simulink model "sandip_MIL_SIL"  (R2019b)
settings: Solver=FixedStepDiscrete  StartTime=0.0  StopTime=16  FixedStep=1  RelTol=1e-3
values from neighbouring files (symbols this model uses):
  Speed = 60.0    [ALS_Project_dd.sldd]    (also in speed_value.m = Simulink.Parameter)
undefined symbols (not defined in the file or in its folder): sigbuilder_block, speed
libraries: simulink x10
settings Model: Creator=Pravin  LastModifiedBy=Pravin
settings ConfigComp: CovEnable=on  RecordCoverage=on  CovMetricSettings=dcmwe  CovModelRefEnable=on

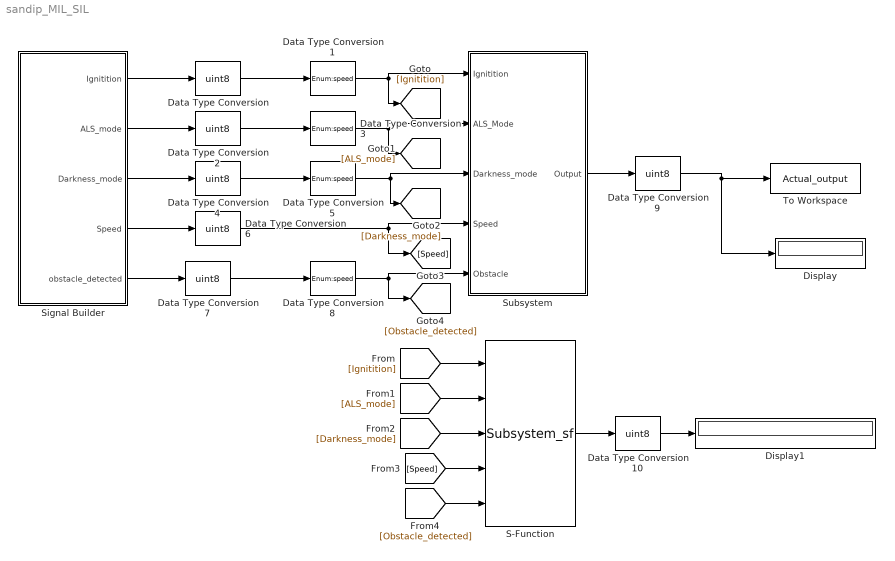
== system sandip_MIL_SIL ==
  Data Type Conversion{,2,4,6..7,9..10} (7 alike) : DataTypeConversion  OutDataTypeStr=uint8
  Data Type Conversion{1,3,5,8} (4 alike) : DataTypeConversion  OutDataTypeStr=Enum:speed
  Display : Display
  Display1 : Display
  S-Function : S-Function  FunctionName=Subsystem_sf  SFunctionDeploymentMode=off  EnableBusSupport=off
  Signal Builder : Subsystem  Tag=STV Subsys  LoadFcn=sigbuilder_block('load',[437.6 153 550.4 359.25 ]);  StartFcn=sigbuilder_block('start');  StopFcn=sigbuilder_block('stop');  ClipboardFcn=sigbuilder_block('clipboard');  mask(Sigbuilder block){tuvar=[0:10]}
      mask help: Simulink:masks:SigbuilderBlock_MD
      mask init:
      | if ~strcmp(get_param(bdroot(gcbh),'SimulationStatus'),'stopped') tuvar = sigbuilder_block('maskInit'); end
      settings: CopyFcn=sigbuilder_block('copy');  DeleteFcn=sigbuilder_block('delete');  ModelCloseFcn=sigbuilder_block('modelClose');  PreSaveFcn=sigbuilder_block('preSave');  PauseFcn=sigbuilder_block('pause');  ContinueFcn=sigbuilder_block('continue');  NameChangeFcn=sigbuilder_block('namechange');  OpenFcn=sigbuilder_block('open',[437.6 153 550.4 359.25 ]);  CloseFcn=sigbuilder_block('close');
      mask Display: plot(0, 0, 100, 100,[2, 2, 32, 32, 2], [68, 8, 8, 68, 68],[32, 2], [38, 38], [32, 19, 2],[53, 60, 44], [32, 17, 17, 2],[16, 16, 31, 31]);txt = getActiveGroup(gcbh);text(2, 100, txt,'verticalAlignment', 'top');
  Subsystem : Subsystem  TreatAsAtomicUnit=on
  To Workspace : ToWorkspace  VariableName=Actual_output  SaveFormat=Timeseries  SampleTime=-1
  wires:
  Signal Builder/1(Ignitition) -> Data Type Conversion/1
  Signal Builder/3(Darkness_mode) -> Data Type Conversion4/1
  Signal Builder/2(ALS_mode) -> Data Type Conversion2/1
  Signal Builder/4(Speed) -> Data Type Conversion6/1
  Signal Builder/5(obstacle_detected) -> Data Type Conversion7/1
  Data Type Conversion/1 -> Data Type Conversion1/1
  Data Type Conversion1/1 -> Subsystem/1(Ignitition), [Ignitition]
  Data Type Conversion2/1 -> Data Type Conversion3/1
  Data Type Conversion4/1 -> Data Type Conversion5/1
  Data Type Conversion5/1 -> [Darkness_mode], Subsystem/3(Darkness_mode)
  Data Type Conversion7/1 -> Data Type Conversion8/1
  Data Type Conversion8/1 -> [Obstacle_detected], Subsystem/5(Obstacle)
  Data Type Conversion9/1 -> Display/1, To Workspace/1
  Data Type Conversion6/1 -> Subsystem/4(Speed), [Speed]
  Data Type Conversion3/1 -> Subsystem/2(ALS_Mode), [ALS_mode]
  Subsystem/1(Output) -> Data Type Conversion9/1
  [Ignitition] -> S-Function/1
  [ALS_mode] -> S-Function/2
  [Darkness_mode] -> S-Function/3
  [Speed] -> S-Function/4
  [Obstacle_detected] -> S-Function/5
  S-Function/1 -> Data Type Conversion10/1
  Data Type Conversion10/1 -> Display1/1

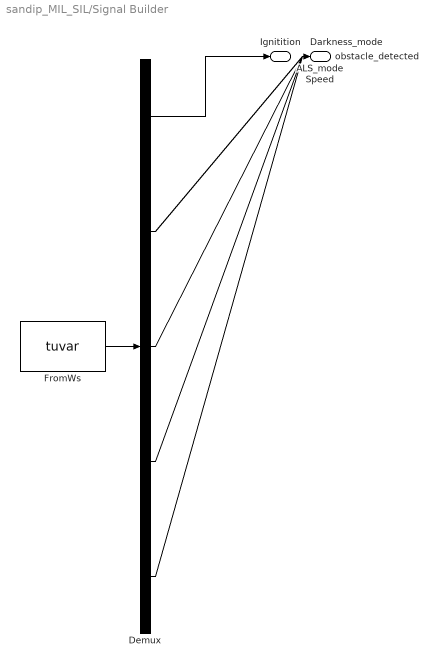
== system sandip_MIL_SIL/Signal Builder ==
  Demux : Demux  Tag=STV Demux  Outputs=5
  FromWs : FromWorkspace  Tag=STV FromWs  VariableName=tuvar  SampleTime=0
      SigBuilderData=|
      | common.afterFinalStr = 'Extrapolate'
      | common.sampleTime = 0
      | dataSet.timeRange = [0 14]
      | dataSet.name = 'Sheet1'
      | sbobj.Name = 'Signal Builder'
      | sbobj.Groups.Name = 'Sheet1'
      | sbobj.Groups.Signals(1).Name = 'Ignitition'
      | sbobj.Groups.Signals(1).XData = [0 1 2 3 4 5 6 7 8 9 10 11 12 13 14]
      | sbobj.Groups.Signals(1).YData = [2 2 2 2 2 2 3 3 2 2 2 2 3 2 2]
      | sbobj.Groups.Signals(2).Name = 'ALS_mode'
      | sbobj.Groups.Signals(2).XData = [0 1 2 3 4 5 6 7 8 9 10 11 12 13 14]
      | sbobj.Groups.Signals(2).YData = [4 4 4 4 4 4 4 5 5 4 4 4 4 5 4]
      | sbobj.Groups.Signals(3).Name = 'Darkness_mode'
      | sbobj.Groups.Signals(3).XData = [0 1 2 3 4 5 6 7 8 9 10 11 12 13 14]
      | sbobj.Groups.Signals(3).YData = [6 6 6 6 6 6 6 6 6 7 6 6 6 6 6]
      | sbobj.Groups.Signals(4).Name = 'Speed'
      | sbobj.Groups.Signals(4).XData = [0 1 2 3 4 5 6 7 8 9 10 11 12 13 14]
      | sbobj.Groups.Signals(4).YData = [29 40 40 30 45 25 40 40 45 30 45 31 30 30 35]
      | sbobj.Groups.Signals(5).Name = 'obstacle_detected'
      | sbobj.Groups.Signals(5).XData = [0 1 2 3 4 5 6 7 8 9 10 11 12 13 14]
      | sbobj.Groups.Signals(5).YData = [10 10 9 10 10 10 10 9 10 10 9 10 10 10 9]
      | sbobj.Groups.TimeRange = [0 14]
  Ignitition : Outport  Tag=STV Outport
  ALS_mode : Outport  Tag=STV Outport  Port=2
  Darkness_mode : Outport  Tag=STV Outport  Port=3
  Speed : Outport  Tag=STV Outport  Port=4
  obstacle_detected : Outport  Tag=STV Outport  Port=5
  wires:
  Demux/1 -> Ignitition/1
  FromWs/1 -> Demux/1
  Demux/2 -> ALS_mode/1
  Demux/3 -> Darkness_mode/1
  Demux/4 -> Speed/1
  Demux/5 -> obstacle_detected/1

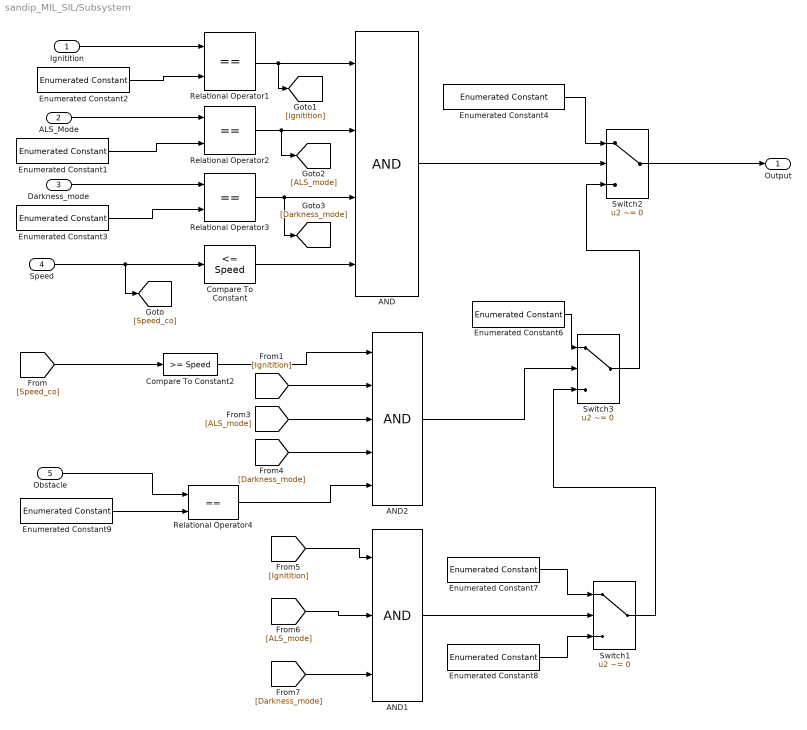
== system sandip_MIL_SIL/Subsystem ==
  Ignitition : Inport
  ALS_Mode : Inport  Port=2
  Darkness_mode : Inport  Port=3
  Speed : Inport  Port=4
  Obstacle : Inport  Port=5
  AND : Logic  Inputs=4  AllPortsSameDT=off  OutDataTypeStr=boolean
  AND1 : Logic  Inputs=3  AllPortsSameDT=off  OutDataTypeStr=boolean
  AND2 : Logic  Inputs=5  AllPortsSameDT=off  OutDataTypeStr=boolean
  Compare To Constant : simulink/Logic and Bit Operations/Compare To Constant  relop=<=  const=Speed  OutDataTypeStr=boolean
  Compare To Constant2 : simulink/Logic and Bit Operations/Compare To Constant  relop=>=  const=Speed  OutDataTypeStr=boolean
  Enumerated Constant1 : simulink/Sources/Enumerated Constant  OutDataTypeStr=Enum:speed  Value=speed.ALS_mode_on  SampleTime=inf
      settings: SourceProductName=Simulink
  Enumerated Constant2 : simulink/Sources/Enumerated Constant  OutDataTypeStr=Enum:speed  Value=speed.Ignitition_on  SampleTime=inf
      settings: SourceProductName=Simulink
  Enumerated Constant3 : simulink/Sources/Enumerated Constant  OutDataTypeStr=Enum:speed  Value=speed.Darkness_mode_on  SampleTime=inf
      settings: SourceProductName=Simulink
  Enumerated Constant4 : simulink/Sources/Enumerated Constant  OutDataTypeStr=Enum:speed  Value=speed.Low_Beam_cornering_light_on  SampleTime=inf
      settings: SourceProductName=Simulink
  Enumerated Constant6 : simulink/Sources/Enumerated Constant  OutDataTypeStr=Enum:speed  Value=speed.High_Beam  SampleTime=inf
      settings: SourceProductName=Simulink
  Enumerated Constant7 : simulink/Sources/Enumerated Constant  OutDataTypeStr=Enum:speed  Value=speed.Low_Beam  SampleTime=inf
      settings: SourceProductName=Simulink
  Enumerated Constant8 : simulink/Sources/Enumerated Constant  OutDataTypeStr=Enum:speed  Value=speed.Headlight_off  SampleTime=inf
      settings: SourceProductName=Simulink
  Enumerated Constant9 : simulink/Sources/Enumerated Constant  OutDataTypeStr=Enum:speed  Value=speed.No_Obstacle_detected  SampleTime=inf
      settings: SourceProductName=Simulink
  Relational Operator{1..4} (4 alike) : RelationalOperator  Operator===  OutDataTypeStr=boolean  RndMeth=Simplest
  Switch1 : Switch  Criteria=u2 ~= 0
  Switch2 : Switch  Criteria=u2 ~= 0
  Switch3 : Switch  Criteria=u2 ~= 0
  Output : Outport
  wires:
  Enumerated Constant1/1 -> Relational Operator2/2
  Switch2/1 -> Output/1
  Relational Operator1/1 -> [Ignitition], AND/1
  Speed/1 -> [Speed_co], Compare To Constant/1
  Enumerated Constant3/1 -> Relational Operator3/2
  Enumerated Constant2/1 -> Relational Operator1/2
  Enumerated Constant4/1 -> Switch2/1
  AND/1 -> Switch2/2
  ALS_Mode/1 -> Relational Operator2/1
  Compare To Constant/1 -> AND/4
  Relational Operator3/1 -> [Darkness_mode], AND/3
  Relational Operator2/1 -> [ALS_mode], AND/2
  Ignitition/1 -> Relational Operator1/1
  Darkness_mode/1 -> Relational Operator3/1
  Compare To Constant2/1 -> AND2/1
  AND2/1 -> Switch3/2
  Enumerated Constant6/1 -> Switch3/1
  Switch3/1 -> Switch2/3
  [Speed_co] -> Compare To Constant2/1
  [Ignitition] -> AND2/2
  [ALS_mode] -> AND2/3
  [Darkness_mode] -> AND2/4
  [Ignitition] -> AND1/1
  [ALS_mode] -> AND1/2
  [Darkness_mode] -> AND1/3
  AND1/1 -> Switch1/2
  Enumerated Constant7/1 -> Switch1/1
  Switch1/1 -> Switch3/3
  Enumerated Constant8/1 -> Switch1/3
  Relational Operator4/1 -> AND2/5
  Obstacle/1 -> Relational Operator4/1
  Enumerated Constant9/1 -> Relational Operator4/2
